simulink model "mod2"  (Simulink 8.1)
settings: Solver=FixedStepDiscrete  StartTime=0.0  StopTime=80e-3  RelTol=1e-3
undefined symbols (not defined in the file): Fs, modctrl
libraries: dspsigops x3, dspsrcs4 x1
settings Model: Creator=amyles  LastModifiedBy=amyles
settings DataIOCC: LimitDataPoints=off  MaxDataPoints=50000
settings OptimizationCC: InlineParams=on
settings DebuggingCC: StrictBusMsg=Warning
settings ModelReferenceCC: ModelReferenceNumInstancesAllowed=Single

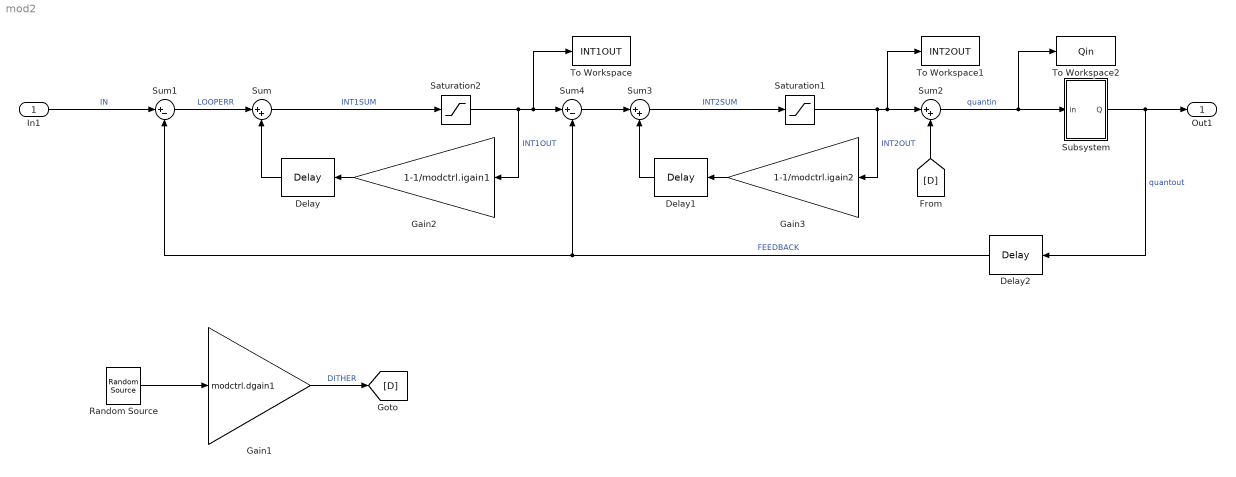
== system mod2 ==
  In1 : Inport
  Delay : dspsigops/Delay  InputProcessing=Inherited (this choice will be removed - see release notes)  dly_unit=Samples  delay=1  ic_detail=off  dif_ic_for_ch=off  dif_ic_for_dly=off  ic=0  reset_popup=None
  Delay1 : dspsigops/Delay  InputProcessing=Inherited (this choice will be removed - see release notes)  dly_unit=Samples  delay=1  ic_detail=off  dif_ic_for_ch=off  dif_ic_for_dly=off  ic=0  reset_popup=None
  Delay2 : dspsigops/Delay  InputProcessing=Inherited (this choice will be removed - see release notes)  dly_unit=Samples  delay=1  ic_detail=off  dif_ic_for_ch=off  dif_ic_for_dly=off  ic=0  reset_popup=None
  Gain1 : Gain  Gain=modctrl.dgain1
      settings: AttributesFormatString=Dither level adjust
  Gain2 : Gain  Gain=1-1/modctrl.igain1
      settings: AttributesFormatString=Integrator leakage
  Gain3 : Gain  Gain=1-1/modctrl.igain2
      settings: AttributesFormatString=Integrator leakage
  Random Source : dspsrcs4/Random Source  SrcType=Uniform  NormMethod=Ziggurat  CltLength=12  MinVal=-1  MaxVal=1  MeanVal=0  VarVal=1  RepMode=Not repeatable  rawSeed=1  IsInherit=off  SampMode=Discrete  SampTime=1/Fs  SampFrame=1  DataType=Double  OutComplex=Real
      settings: AttributesFormatString=Dither source
  Saturation1 : Saturate  UpperLimit=modctrl.isat2  LowerLimit=-(modctrl.isat2)
  Saturation2 : Saturate  UpperLimit=modctrl.isat1  LowerLimit=-(modctrl.isat1)
  Subsystem : Subsystem
      settings: AttributesFormatString=1-bit quantiser
  Sum : Sum  Inputs=|++
      settings: AttributesFormatString=Integrator summer
  Sum1 : Sum  Inputs=|+-
      settings: AttributesFormatString=Modulator input\nloop servo error (input - fbk)
  Sum2 : Sum  Inputs=|++
  Sum3 : Sum  Inputs=|++
      settings: AttributesFormatString=Integrator summer
  Sum4 : Sum  Inputs=|+-
  To Workspace : ToWorkspace  VariableName=INT1OUT  SampleTime=-1
  To Workspace1 : ToWorkspace  VariableName=INT2OUT  SampleTime=-1
  To Workspace2 : ToWorkspace  VariableName=Qin  SampleTime=-1
  Out1 : Outport
  wires:
  Delay/1 -> Sum/2
  Sum/1 -> Saturation2/1  "INT1SUM"
  Sum1/1 -> Sum/1  "LOOPERR"
  Delay2/1 -> Sum1/2, Sum4/2  "FEEDBACK"
  In1/1 -> Sum1/1  "IN"
  Sum2/1 -> Subsystem/1(in), To Workspace2/1  "quantin"
  Gain2/1 -> Delay/1
  Subsystem/1(Q) -> Delay2/1, Out1/1  "quantout"
  Delay1/1 -> Sum3/2
  Sum3/1 -> Saturation1/1  "INT2SUM"
  Sum4/1 -> Sum3/1
  Gain3/1 -> Delay1/1
  Saturation1/1 -> Gain3/1, Sum2/1, To Workspace1/1  "INT2OUT"
  Saturation2/1 -> Gain2/1, Sum4/1, To Workspace/1  "INT1OUT"
  Random Source/1 -> Gain1/1
  [D] -> Sum2/2
  Gain1/1 -> [D]  "DITHER"

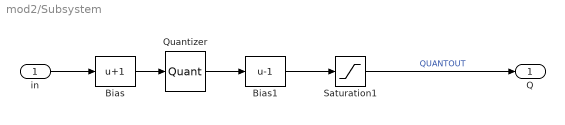
== system mod2/Subsystem ==
  in : Inport
  Bias : Bias  Bias=1
      settings: AttributesFormatString=Need offset to give\nMID-RISE quantiser
  Bias1 : Bias  Bias=-1
      settings: AttributesFormatString=1
  Quantizer : Quantizer  QuantizationInterval=2  LinearizeAsGain=off
  Saturation1 : Saturate  UpperLimit=1  LowerLimit=-1
      settings: AttributesFormatString=Limit quantiser\noutput to +/-1
  Q : Outport
  wires:
  Bias/1 -> Quantizer/1
  Quantizer/1 -> Bias1/1
  Bias1/1 -> Saturation1/1
  in/1 -> Bias/1
  Saturation1/1 -> Q/1  "QUANTOUT"
